simulink model "tankmeasure"  (R2015b)
settings: Solver=VariableStepAuto  StartTime=0.0  StopTime=50.0  RelTol=1e-3
settings Model: Creator=PC  LastModifiedBy=PC

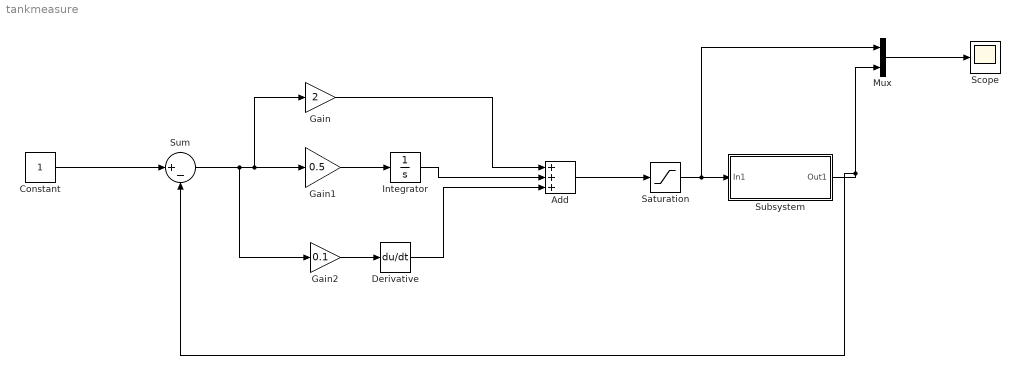
== system tankmeasure ==
  Add : Sum  Inputs=+++
  Constant : Constant
  Derivative : Derivative
  Gain : Gain  Gain=2
  Gain1 : Gain  Gain=0.5
  Gain2 : Gain  Gain=0.1
  Integrator : Integrator
  Mux : Mux  Inputs=2
  Saturation : Saturate  UpperLimit=5  LowerLimit=0
  Scope : Scope
  Subsystem : Subsystem
  Sum : Sum  Inputs=|+-
  wires:
  Constant/1 -> Sum/1
  Add/1 -> Saturation/1
  Gain1/1 -> Integrator/1
  Gain/1 -> Add/1
  Gain2/1 -> Derivative/1
  Sum/1 -> Gain/1, Gain1/1, Gain2/1
  Saturation/1 -> Mux/1, Subsystem/1(In1)
  Derivative/1 -> Add/3
  Integrator/1 -> Add/2
  Subsystem/1(Out1) -> Sum/2, Mux/2
  Mux/1 -> Scope/1

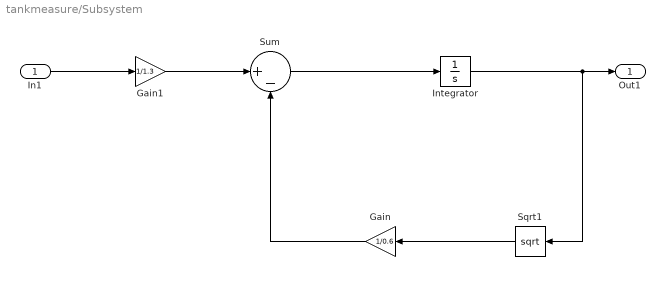
== system tankmeasure/Subsystem ==
  In1 : Inport
  Gain : Gain  Gain=1/0.6
  Gain1 : Gain  Gain=1/1.3
  Integrator : Integrator
  Sqrt1 : Sqrt  SaturateOnIntegerOverflow=on
  Sum : Sum  Inputs=|+-
  Out1 : Outport
  wires:
  Sum/1 -> Integrator/1
  Gain1/1 -> Sum/1
  In1/1 -> Gain1/1
  Integrator/1 -> Sqrt1/1, Out1/1
  Sqrt1/1 -> Gain/1
  Gain/1 -> Sum/2
